simulink model "cmult_core"  (R2013a)
settings: Solver=ode45  StartTime=0.0  StopTime=10.0  RelTol=1e-3
libraries: xbsIndex_r4 x2035, casper_library_misc x116, casper_library_multipliers x36
(part 1 of 23)
settings Model: Creator=jack  LastModifiedBy=jack
settings OptimizationCC: ExpressionDepthLimit=2147483647

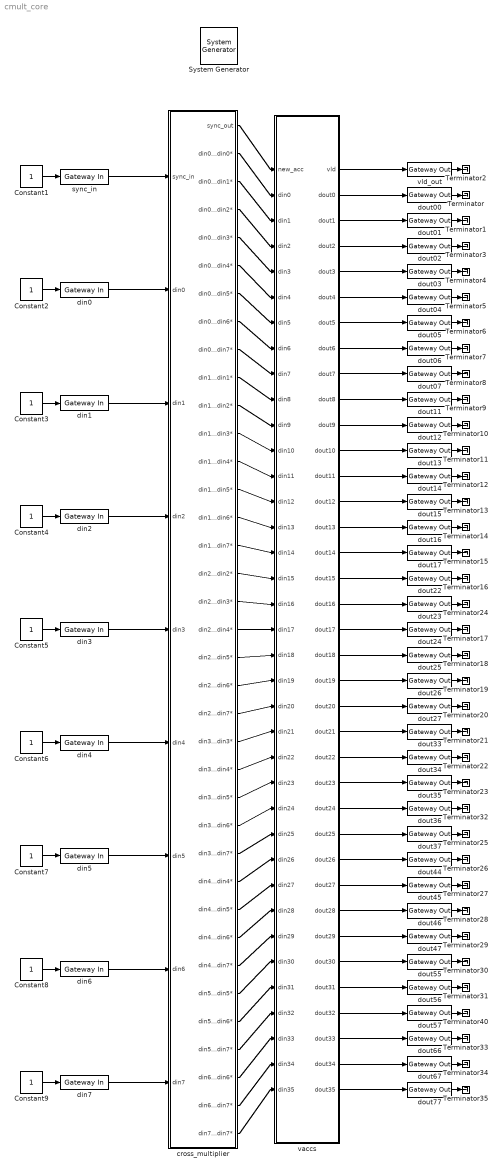
== system cmult_core ==
  " System Generator" : xbsIndex_r4/ System Generator  Tag=genX  xilinxfamily=virtex6  part=xc6vsx475t  speed=-1  package=ff1759  synthesis_tool=XST  clock_wrapper=Clock Enables  directory=./cmult_core  proj_type=Project Navigator  Synth_file=XST Defaults  Impl_file=ISE Defaults  testbench=off  simulink_period=1  sysclk_period=3.2  dcm_input_clock_period=10  incr_netlist=off  trim_vbits=Everywhere in SubSystem  dbl_ovrd=According to Block Masks  core_generation=According to Block Masks  run_coregen=off  deprecated_control=off  eval_field=0  block_type=sysgen
  Constant{1..9} (9 alike) : Constant
  Terminator{,1..35,40} (37 alike) : Terminator
  cross_multiplier : Subsystem  mask(cross_multiplier){streams=8, aggregation=1, bit_width_in=8, binary_point_in=7, bit_width_out=17, binary_point_out=14, mult_latency=3, add_latency=1, overflow=Wrap, quantisation=Truncate, conv_latency=0}
      mask prompts: streams "Number input streams"; aggregation "Aggregation per stream"; bit_width_in "Bit width in"; binary_point_in "Binary point in"; bit_width_out "Bit width out"; binary_point_out "Binary point out"; mult_latency "Multiplier latency"; add_latency "Adder latency"; overflow "Overflow behaviour"; quantisation "Quantisation behaviour"; conv_latency "Bit width conversion latency"
      mask help: Cross multiplies aggregated complex input streams.
      mask init:
      | cross_multiplier_init(gcb, ...
      |     'streams', streams, ...
      |     'aggregation', aggregation, ...
      |     'bit_width_in', bit_width_in, ...
      |     'binary_point_in', binary_point_in, ...
      |     'bit_width_out', bit_width_out, ...
      |     'binary_point_out', binary_point_out, ...
      |     'mult_latency', mult_latency, ...
      |     'add_latency', add_latency, ...
      |     'overflow', overflow, ...
      |     'quantisation', quantisation, ...
      |     'conv_latency', conv_latency);
      mask TypeOptions overflow: Wrap | Saturate | Error
      mask TypeOptions quantisation: Truncate | Round  (unbiased: +/- Inf) | Round  (unbiased: even values)
  din{0..7} (8 alike) : xbsIndex_r4/Gateway In  gui_display_data_type=Fixed-point  arith_type=Unsigned  n_bits=16  bin_pt=0  preci_type=Single  exp_width=8  frac_width=24  quantization="Round  (unbiased: +/- Inf)"  overflow=Saturate  period=1  dbl_ovrd=off  timing_constraint=None  locs_specified=off  LOCs={}  UseAsADC=off  ADCChannel='1'  inherit_from_input=off  hdl_port=on  block_type=gatewayin
  dout00 : xbsIndex_r4/Gateway Out  inherit_from_input=off  hdl_port=on  timing_constraint=None  locs_specified=off  LOCs={}  UseAsDAC=off  DACChannel='1'  block_type=gatewayout
  dout01 : xbsIndex_r4/Gateway Out  inherit_from_input=off  hdl_port=on  timing_constraint=None  locs_specified=off  LOCs={}  UseAsDAC=off  DACChannel='1'  block_type=gatewayout
  dout02 : xbsIndex_r4/Gateway Out  inherit_from_input=off  hdl_port=on  timing_constraint=None  locs_specified=off  LOCs={}  UseAsDAC=off  DACChannel='1'  block_type=gatewayout
  dout03 : xbsIndex_r4/Gateway Out  inherit_from_input=off  hdl_port=on  timing_constraint=None  locs_specified=off  LOCs={}  UseAsDAC=off  DACChannel='1'  block_type=gatewayout
  dout04 : xbsIndex_r4/Gateway Out  inherit_from_input=off  hdl_port=on  timing_constraint=None  locs_specified=off  LOCs={}  UseAsDAC=off  DACChannel='1'  block_type=gatewayout
  dout05 : xbsIndex_r4/Gateway Out  inherit_from_input=off  hdl_port=on  timing_constraint=None  locs_specified=off  LOCs={}  UseAsDAC=off  DACChannel='1'  block_type=gatewayout
  dout06 : xbsIndex_r4/Gateway Out  inherit_from_input=off  hdl_port=on  timing_constraint=None  locs_specified=off  LOCs={}  UseAsDAC=off  DACChannel='1'  block_type=gatewayout
  dout07 : xbsIndex_r4/Gateway Out  inherit_from_input=off  hdl_port=on  timing_constraint=None  locs_specified=off  LOCs={}  UseAsDAC=off  DACChannel='1'  block_type=gatewayout
  dout{11..17,22..27,33..37,44..47,55..57,66..67,77} (28 alike) : xbsIndex_r4/Gateway Out  inherit_from_input=off  hdl_port=on  timing_constraint=None  locs_specified=off  LOCs={}  UseAsDAC=off  DACChannel='1'  block_type=gatewayout
  sync_in : xbsIndex_r4/Gateway In  gui_display_data_type=Boolean  arith_type=Boolean  n_bits=16  bin_pt=14  preci_type=Single  exp_width=8  frac_width=24  quantization="Round  (unbiased: +/- Inf)"  overflow=Saturate  period=1  dbl_ovrd=off  timing_constraint=None  locs_specified=off  LOCs={}  UseAsADC=off  ADCChannel='1'  inherit_from_input=off  hdl_port=on  block_type=gatewayin
  vaccs : Subsystem  mask{vacc_len=1024}
      mask prompts: vacc_len "vacc length"
  vld_out : xbsIndex_r4/Gateway Out  inherit_from_input=off  hdl_port=on  timing_constraint=None  locs_specified=off  LOCs={}  UseAsDAC=off  DACChannel='1'  block_type=gatewayout
  wires:
  Constant1/1 -> sync_in/1
  Constant2/1 -> din0/1
  dout00/1 -> Terminator/1
  vld_out/1 -> Terminator2/1
  sync_in/1 -> cross_multiplier/1(sync_in)
  din0/1 -> cross_multiplier/2(din0)
  Constant3/1 -> din1/1
  Constant4/1 -> din2/1
  Constant5/1 -> din3/1
  Constant6/1 -> din4/1
  Constant7/1 -> din5/1
  Constant8/1 -> din6/1
  Constant9/1 -> din7/1
  din7/1 -> cross_multiplier/9(din7)
  din4/1 -> cross_multiplier/6(din4)
  din2/1 -> cross_multiplier/4(din2)
  din6/1 -> cross_multiplier/8(din6)
  din1/1 -> cross_multiplier/3(din1)
  din5/1 -> cross_multiplier/7(din5)
  din3/1 -> cross_multiplier/5(din3)
  dout01/1 -> Terminator1/1
  dout02/1 -> Terminator3/1
  dout03/1 -> Terminator4/1
  dout05/1 -> Terminator6/1
  dout06/1 -> Terminator7/1
  dout07/1 -> Terminator8/1
  dout11/1 -> Terminator9/1
  dout12/1 -> Terminator10/1
  dout13/1 -> Terminator11/1
  dout14/1 -> Terminator12/1
  dout16/1 -> Terminator14/1
  dout17/1 -> Terminator15/1
  dout22/1 -> Terminator16/1
  dout23/1 -> Terminator24/1
  dout24/1 -> Terminator17/1
  dout25/1 -> Terminator18/1
  dout26/1 -> Terminator19/1
  dout33/1 -> Terminator21/1
  dout34/1 -> Terminator22/1
  dout35/1 -> Terminator23/1
  dout36/1 -> Terminator32/1
  dout37/1 -> Terminator25/1
  dout44/1 -> Terminator26/1
  dout45/1 -> Terminator27/1
  dout47/1 -> Terminator29/1
  dout55/1 -> Terminator30/1
  dout56/1 -> Terminator31/1
  dout57/1 -> Terminator40/1
  dout66/1 -> Terminator33/1
  dout67/1 -> Terminator34/1
  dout77/1 -> Terminator35/1
  dout15/1 -> Terminator13/1
  dout46/1 -> Terminator28/1
  dout27/1 -> Terminator20/1
  dout04/1 -> Terminator5/1
  cross_multiplier/1(sync_out) -> vaccs/1(new_acc)
  cross_multiplier/12(din1_x_din3*) -> vaccs/12(din10)
  cross_multiplier/6(din0_x_din4*) -> vaccs/6(din4)
  cross_multiplier/23(din3_x_din3*) -> vaccs/23(din21)
  cross_multiplier/32(din5_x_din5*) -> vaccs/32(din30)
  cross_multiplier/9(din0_x_din7*) -> vaccs/9(din7)
  cross_multiplier/25(din3_x_din5*) -> vaccs/25(din23)
  cross_multiplier/20(din2_x_din5*) -> vaccs/20(din18)
  cross_multiplier/4(din0_x_din2*) -> vaccs/4(din2)
  cross_multiplier/8(din0_x_din6*) -> vaccs/8(din6)
  cross_multiplier/19(din2_x_din4*) -> vaccs/19(din17)
  cross_multiplier/26(din3_x_din6*) -> vaccs/26(din24)
  cross_multiplier/21(din2_x_din6*) -> vaccs/21(din19)
  cross_multiplier/37(din7_x_din7*) -> vaccs/37(din35)
  cross_multiplier/33(din5_x_din6*) -> vaccs/33(din31)
  cross_multiplier/7(din0_x_din5*) -> vaccs/7(din5)
  cross_multiplier/3(din0_x_din1*) -> vaccs/3(din1)
  cross_multiplier/15(din1_x_din6*) -> vaccs/15(din13)
  cross_multiplier/35(din6_x_din6*) -> vaccs/35(din33)
  cross_multiplier/14(din1_x_din5*) -> vaccs/14(din12)
  cross_multiplier/18(din2_x_din3*) -> vaccs/18(din16)
  cross_multiplier/24(din3_x_din4*) -> vaccs/24(din22)
  cross_multiplier/10(din1_x_din1*) -> vaccs/10(din8)
  cross_multiplier/5(din0_x_din3*) -> vaccs/5(din3)
  cross_multiplier/16(din1_x_din7*) -> vaccs/16(din14)
  cross_multiplier/22(din2_x_din7*) -> vaccs/22(din20)
  cross_multiplier/34(din5_x_din7*) -> vaccs/34(din32)
  cross_multiplier/28(din4_x_din4*) -> vaccs/28(din26)
  cross_multiplier/31(din4_x_din7*) -> vaccs/31(din29)
  cross_multiplier/11(din1_x_din2*) -> vaccs/11(din9)
  cross_multiplier/2(din0_x_din0*) -> vaccs/2(din0)
  cross_multiplier/27(din3_x_din7*) -> vaccs/27(din25)
  cross_multiplier/30(din4_x_din6*) -> vaccs/30(din28)
  cross_multiplier/17(din2_x_din2*) -> vaccs/17(din15)
  cross_multiplier/36(din6_x_din7*) -> vaccs/36(din34)
  cross_multiplier/13(din1_x_din4*) -> vaccs/13(din11)
  cross_multiplier/29(din4_x_din5*) -> vaccs/29(din27)
  vaccs/1(vld) -> vld_out/1
  vaccs/2(dout0) -> dout00/1
  vaccs/3(dout1) -> dout01/1
  vaccs/4(dout2) -> dout02/1
  vaccs/5(dout3) -> dout03/1
  vaccs/6(dout4) -> dout04/1
  vaccs/7(dout5) -> dout05/1
  vaccs/8(dout6) -> dout06/1
  vaccs/9(dout7) -> dout07/1
  vaccs/10(dout8) -> dout11/1
  vaccs/11(dout9) -> dout12/1
  vaccs/12(dout10) -> dout13/1
  vaccs/13(dout11) -> dout14/1
  vaccs/14(dout12) -> dout15/1
  vaccs/15(dout13) -> dout16/1
  vaccs/16(dout14) -> dout17/1
  vaccs/17(dout15) -> dout22/1
  vaccs/18(dout16) -> dout23/1
  vaccs/19(dout17) -> dout24/1
  vaccs/20(dout18) -> dout25/1
  vaccs/21(dout19) -> dout26/1
  vaccs/22(dout20) -> dout27/1
  vaccs/23(dout21) -> dout33/1
  vaccs/24(dout22) -> dout34/1
  vaccs/25(dout23) -> dout35/1
  vaccs/26(dout24) -> dout36/1
  vaccs/27(dout25) -> dout37/1
  vaccs/28(dout26) -> dout44/1
  vaccs/29(dout27) -> dout45/1
  vaccs/30(dout28) -> dout46/1
  vaccs/31(dout29) -> dout47/1
  vaccs/32(dout30) -> dout55/1
  vaccs/33(dout31) -> dout56/1
  vaccs/34(dout32) -> dout57/1
  vaccs/35(dout33) -> dout66/1
  vaccs/36(dout34) -> dout67/1
  vaccs/37(dout35) -> dout77/1
